simulink model "S_new"  (R2019a)
settings: Solver=VariableStepAuto  StartTime=0.0  StopTime=10.0  RelTol=1e-3
undefined symbols (not defined in the file or in its folder): N1, N2
settings Model: Creator=rache  LastModifiedBy=rache

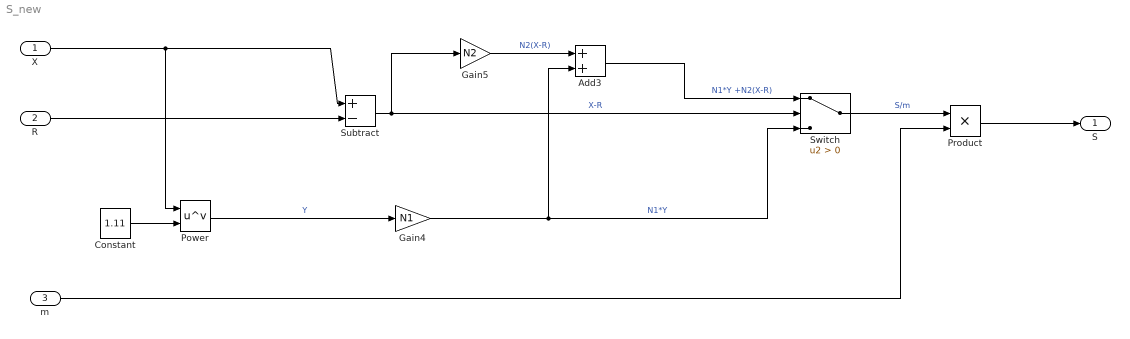
== system S_new ==
  X : Inport
  R : Inport  Port=2
  "m " : Inport  Port=3
  Add3 : Sum
  Constant : Constant  Value=1.11
  Gain4 : Gain  Gain=N1
  Gain5 : Gain  Gain=N2
  Power : Math  Operator=pow  SaturateOnIntegerOverflow=on
  Product : Product
  Subtract : Sum  Inputs=+-
  Switch : Switch  Criteria=u2 > Threshold
  S : Outport
  wires:
  R/1 -> Subtract/2
  Gain4/1 -> Add3/2, Switch/3  "N1*Y"
  Add3/1 -> Switch/1  "N1*Y +N2(X-R)"
  Constant/1 -> Power/2
  X/1 -> Power/1, Subtract/1
  Power/1 -> Gain4/1  "Y"
  Gain5/1 -> Add3/1  "N2(X-R)"
  Subtract/1 -> Gain5/1, Switch/2  "X-R"
  Switch/1 -> Product/1  "S/m"
  "m "/1 -> Product/2
  Product/1 -> S/1
